simulink model "stretch_reflex"  (R2022a)
settings: Solver=VariableStepAuto  StartTime=0.0  StopTime=1  RelTol=1e-3
model workspace: external: MATLAB File stretch_reflex_parameters.m (data not in the file)
values from neighbouring files (symbols this model uses):
  B = 2    [stretch_reflex_parameters.m]
  beta = 156.1922167275855    (= 156.192216728)    [stretch_reflex_parameters.m]    (also in stretch_reflex_stability.m = 100)
  eta = 5    [stretch_reflex_parameters.m]
  J = 0.1    [stretch_reflex_parameters.m]
  k = 50    [stretch_reflex_parameters.m]
  tau = 0.0033333333333333335    (= 0.00333333333333)    [stretch_reflex_parameters.m]
  Td = 0.02    [stretch_reflex_parameters.m]    (also in stretch_reflex_stability.m)
settings Model: Creator=bigba  LastModifiedBy=alessandromastrofini
settings DebuggingCC: UnconnectedInputMsg=warning  UnconnectedOutputMsg=warning  UnconnectedLineMsg=warning
settings RTWCC: DLArmComputeVersion=19.05
settings ConfigComp: CovHTMLOptions=-sRT=1 -sVT=0 -aTS=1 -agT=1 -bRG=1 -bTC=1 -hTR=0 -nFC=0 -nFD=1 -scm=1 -bcm=1 -xEv=0 -xEM=0 -req=1  CovEnableCumulative=off

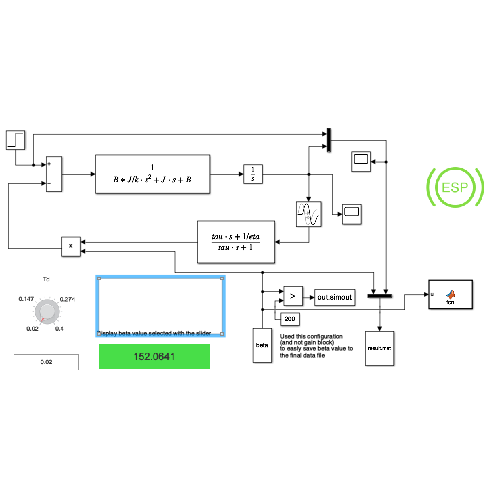
[thumbnail: Simulink's stored preview of the top-level diagram]
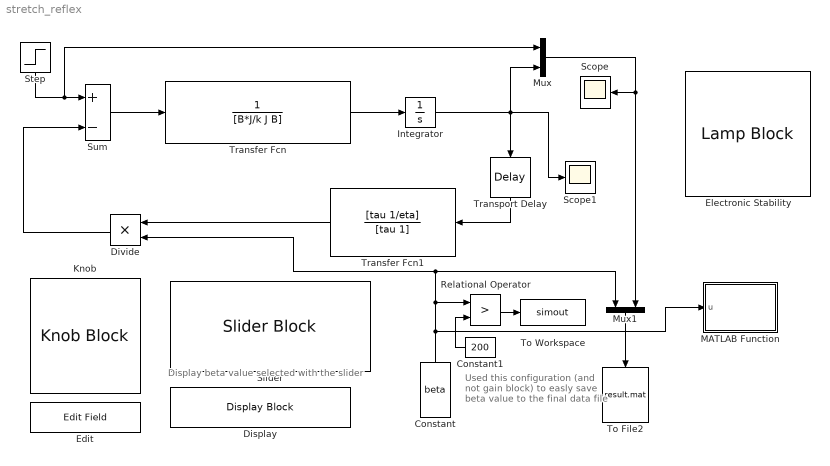
== system stretch_reflex ==
  note: Used this configuration (and not gain block)
      | to easly save beta value to the final data file
  note: Display beta value selected with the slider
  Constant : Constant  Value=beta
  Constant1 : Constant  Value=200
  Display : DisplayBlock  LabelPosition=Hide  Transparency=1  Opacity=0.9
  Divide : Product  Inputs=**
  Edit : EditField  LabelPosition=Hide  ShowInitialText=on  Alignment=Center
  Electronic Stability : LampBlock  LabelPosition=Hide  Icon=ElectronicStability
  Integrator : Integrator
  Knob : KnobBlock  ScaleMin=0.02  ScaleMax=0.4
  MATLAB Function : MATLAB Function  TreatAsAtomicUnit=on
  Mux : Mux  Inputs=2
  Mux1 : Mux  Inputs=2
  Relational Operator : RelationalOperator  Operator=>  OutDataTypeStr=boolean  RndMeth=Simplest  InputSameDT=off
  Scope : Scope
  Scope1 : Scope
  Slider : SliderBlock  ScaleMin=50  ScaleMax=250  TickInterval=50
  Step : Step  Time=0.1  After=5  SampleTime=0
  Sum : Sum  Inputs=+-
  To File2 : ToFile  Filename=result.mat  MatrixName=stretch_reflex_result  SaveFormat=Timeseries
  To Workspace : ToWorkspace  VariableName=simout  SaveFormat=Timeseries  SampleTime=-1
  Transfer Fcn : TransferFcn  Denominator=[B*J/k J B]
  Transfer Fcn1 : TransferFcn  Numerator=[tau 1/eta]  Denominator=[tau 1]
  Transport Delay : TransportDelay  DelayTime=Td  InitialOutput=0.01545652198791504
  wires:
  Sum/1 -> Transfer Fcn/1
  Transfer Fcn/1 -> Integrator/1
  Integrator/1 -> Scope1/1, Transport Delay/1, Mux/2
  Transport Delay/1 -> Transfer Fcn1/1
  Mux/1 -> Mux1/2, Scope/1
  Transfer Fcn1/1 -> Divide/1
  Mux1/1 -> To File2/1
  Constant/1 -> Mux1/1, Divide/2, Relational Operator/1, MATLAB Function/1(u)
  Divide/1 -> Sum/2
  Step/1 -> Mux/1, Sum/1
  Constant1/1 -> Relational Operator/2
  Relational Operator/1 -> To Workspace/1

== matlab function stretch_reflex/MATLAB Function ==
  data: u input
function fcn(u)

if u>200
set_param('stretch_reflex/Display','BackgroundColor','red');

else
set_param('stretch_reflex/Display','BackgroundColor','green');
end
